simulink model "part1_done"  (R2024b)
settings: Solver=VariableStepAuto  StartTime=0.0  StopTime=1000  RelTol=1e-3

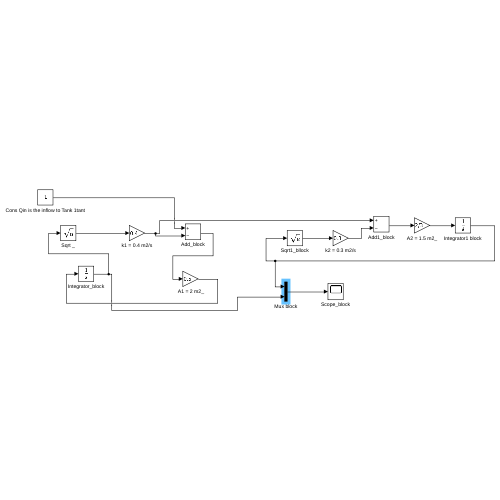
[thumbnail: Simulink's stored preview of the top-level diagram]
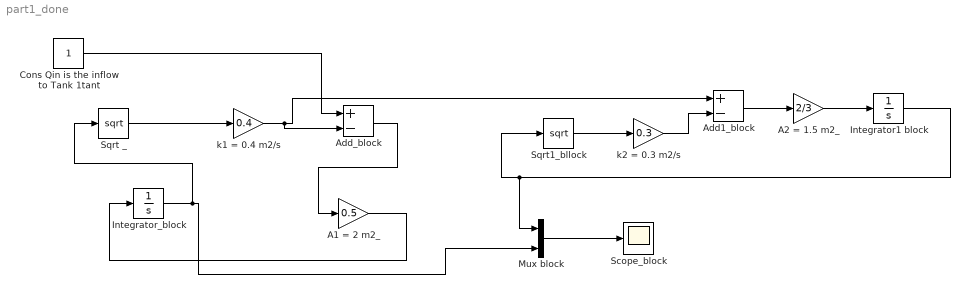
== system part1_done ==
  " A1 = 2 m2_" : Gain  Gain=0.5
  A2 = 1.5 m2_ : Gain  Gain=2/3
  Add1_block : Sum  Inputs=+-
  Add_block : Sum  Inputs=+-
  Cons Qin is the inflow to Tank 1tant : Constant
  Integrator1 block : Integrator
  Integrator_block : Integrator
  Mux block : Mux  Inputs=2
  Scope_block : Scope
  Sqrt _ : Sqrt
  Sqrt1_bllock : Sqrt
  k1 = 0.4 m2/s : Gain  Gain=0.4
  k2 = 0.3 m2/s : Gain  Gain=0.3
  wires:
  Cons Qin is the inflow to Tank 1tant/1 -> Add_block/1
  Add_block/1 -> " A1 = 2 m2_"/1
  " A1 = 2 m2_"/1 -> Integrator_block/1
  Sqrt1_bllock/1 -> k2 = 0.3 m2/s/1
  k2 = 0.3 m2/s/1 -> Add1_block/2
  Add1_block/1 -> A2 = 1.5 m2_/1
  A2 = 1.5 m2_/1 -> Integrator1 block/1
  Integrator1 block/1 -> Mux block/1, Sqrt1_bllock/1
  Mux block/1 -> Scope_block/1
  Integrator_block/1 -> Sqrt _/1, Mux block/2
  Sqrt _/1 -> k1 = 0.4 m2/s/1
  k1 = 0.4 m2/s/1 -> Add_block/2, Add1_block/1
